simulink model "heave_surge_tfns"  (R2018b)
settings: Solver=VariableStepAuto  StartTime=0.0  StopTime=10.0  RelTol=1e-3
undefined symbols (not defined in the file or in its folder): tfheave_04den, tfheave_04num, tfsurge_04den, tfsurge_04num
libraries: slctrlblks x1
settings Model: Creator=user  LastModifiedBy=user

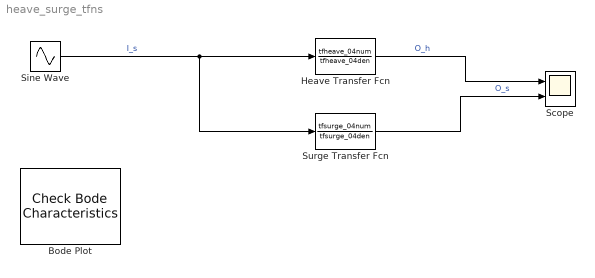
== system heave_surge_tfns ==
  Bode Plot : slctrlblks/Model Verification/Check Bode  Characteristics  InstantiateOnLoad=on  SaveOperatingPoints=off  LinearizationIOs={'/Sine Wave', 1, 'in', 'off', '';'/Surge Transfer Fcn', 1, 'out', 'on', ''}  LinearizeAt=SnapshotTimes  SnapshotTimes=[0]  TriggerType=rising  SampleTime=auto  RateConversionMethod=zoh  PreWarpFreq=10  UseExactDelayModel=off  UseFullBlockNameLabels=off  UseBusSignalLabels=off  enabled=on  stopWhenAssertionFail=off  export=off  ViewDlgPos=[623.4 165 509.6 389.6]  OpenViewOnLoad=off  LaunchViewOnOpen=off  FrequencyUnits=rad/s  MagnitudeUnits=dB  PhaseUnits=deg  TimeUnits=seconds  EnableUpperBound=off  UpperBoundFrequencies=[]  UpperBoundMagnitudes=[]  EnableLowerBound=off  LowerBoundFrequencies=[]  LowerBoundMagnitudes=[]
      settings: SourceProductName=Simulink Control Design  SaveToWorkspace=on  SaveName=Surge
  Heave Transfer Fcn : TransferFcn  Numerator=tfheave_04num  Denominator=tfheave_04den
  Scope : Scope  NumInputPorts=2
  Sine Wave : Sin  Amplitude=100  Frequency=2  SampleTime=0
  Surge Transfer Fcn : TransferFcn  Numerator=tfsurge_04num  Denominator=tfsurge_04den
  wires:
  Sine Wave/1 -> Surge Transfer Fcn/1, Heave Transfer Fcn/1  "I_s"
  Heave Transfer Fcn/1 -> Scope/1  "O_h"
  Surge Transfer Fcn/1 -> Scope/2  "O_s"
